simulink model "BitBlocks_model_2019v"  (R2022b)
settings: Solver=VariableStepAuto  StartTime=0.0  StopTime=10.0  RelTol=1e-3
libraries: simulink x6
settings Model: Creator=Brigosha_Guest  LastModifiedBy=Brigosha_Guest

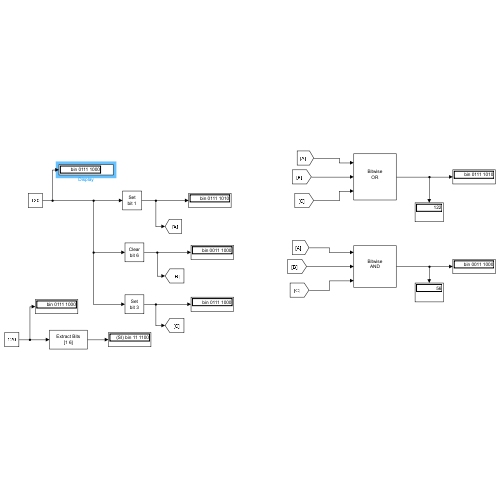
[thumbnail: Simulink's stored preview of the top-level diagram]
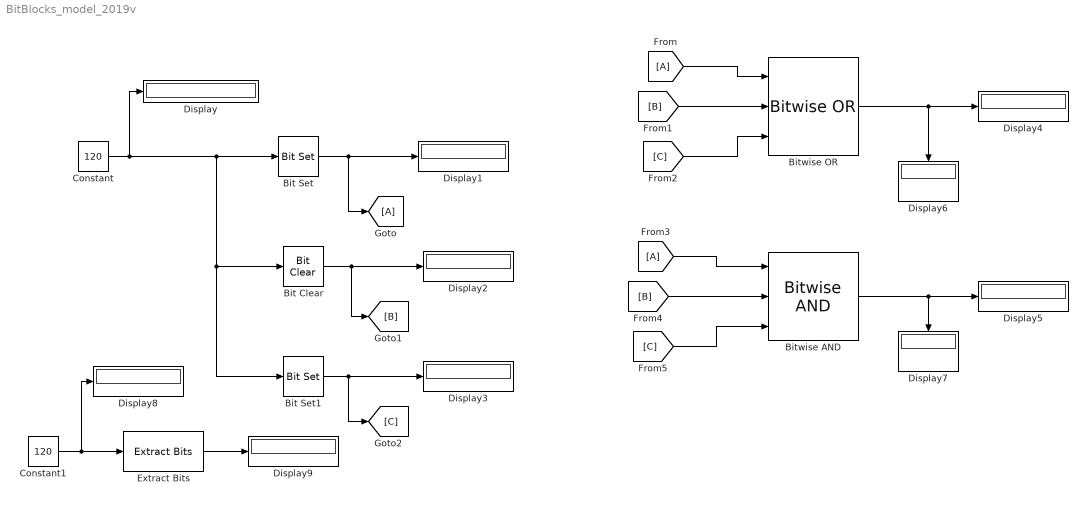
== system BitBlocks_model_2019v ==
  Bit Clear : simulink/Logic and Bit Operations/Bit Clear  iBit=6
  Bit Set : simulink/Logic and Bit Operations/Bit Set  iBit=1
  Bit Set1 : simulink/Logic and Bit Operations/Bit Set  iBit=3
  Bitwise AND : simulink/Logic and Bit Operations/Bitwise Operator  logicop=AND  UseBitMask=off  NumInputPorts=3  BitMask=bin2dec('11011001')  BitMaskRealWorld=Stored Integer
      settings: LibrarySourceBlock=|
      | simulink/Quick Insert/Logic and Bit
      | Operations/Bitwise AND
  Bitwise OR : simulink/Logic and Bit Operations/Bitwise Operator  logicop=OR  UseBitMask=off  NumInputPorts=3  BitMask=bin2dec('11011001')  BitMaskRealWorld=Stored Integer
      settings: LibrarySourceBlock=|
      | simulink/Quick Insert/Logic and Bit
      | Operations/Bitwise OR
  Constant : Constant  Value=120  OutDataTypeStr=int8
  Constant1 : Constant  Value=120  OutDataTypeStr=int8
  Display{,1..9} (10 alike) : Display
      Display settings: Format=binary (Stored Integer)
      Display1 settings: Format=binary (Stored Integer)
      Display2 settings: Format=binary (Stored Integer)
      Display3 settings: Format=binary (Stored Integer)
      Display4 settings: Format=binary (Stored Integer)
      Display5 settings: Format=binary (Stored Integer)
      Display6 settings: Format=decimal (Stored Integer)
      Display7 settings: Format=decimal (Stored Integer)
      Display8 settings: Format=binary (Stored Integer)
      Display9 settings: Format=binary (Stored Integer)
  Extract Bits : simulink/Logic and Bit Operations/Extract Bits  bitsToExtract=Range of bits  numBits=8  bitIdxRange=[1 6]  outScalingMode=Preserve fixed-point scaling
  From : From
  From3 : From
  Goto : Goto
  wires:
  Constant/1 -> Display/1, Bit Set1/1, Bit Clear/1, Bit Set/1
  Bit Set/1 -> Goto/1, Display1/1
  Bit Set1/1 -> [C], Display3/1
  Bit Clear/1 -> [B], Display2/1
  Bitwise OR/1 -> Display4/1, Display6/1
  From/1 -> Bitwise OR/1
  [B] -> Bitwise OR/2
  [C] -> Bitwise OR/3
  [C] -> Bitwise AND/3
  [B] -> Bitwise AND/2
  From3/1 -> Bitwise AND/1
  Bitwise AND/1 -> Display7/1, Display5/1
  Constant1/1 -> Display8/1, Extract Bits/1
  Extract Bits/1 -> Display9/1
